simulink model "TurtlebotClosedLoop_template"  (R2023b)
settings: Solver=VariableStepAuto  StartTime=0.0  StopTime=150  MaxStep=0.1  RelTol=1e-3
undefined symbols (not defined in the file): q0
libraries: slpidlib x2, robotcorelib x1, robotmobilelib x1
settings Model: Creator=tpoggi  LastModifiedBy=jonpe

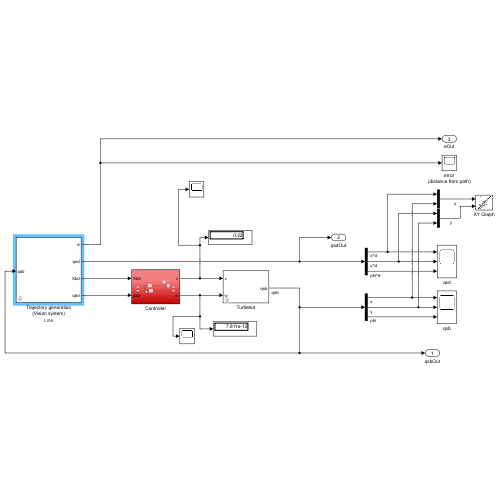
[thumbnail: Simulink's stored preview of the top-level diagram]
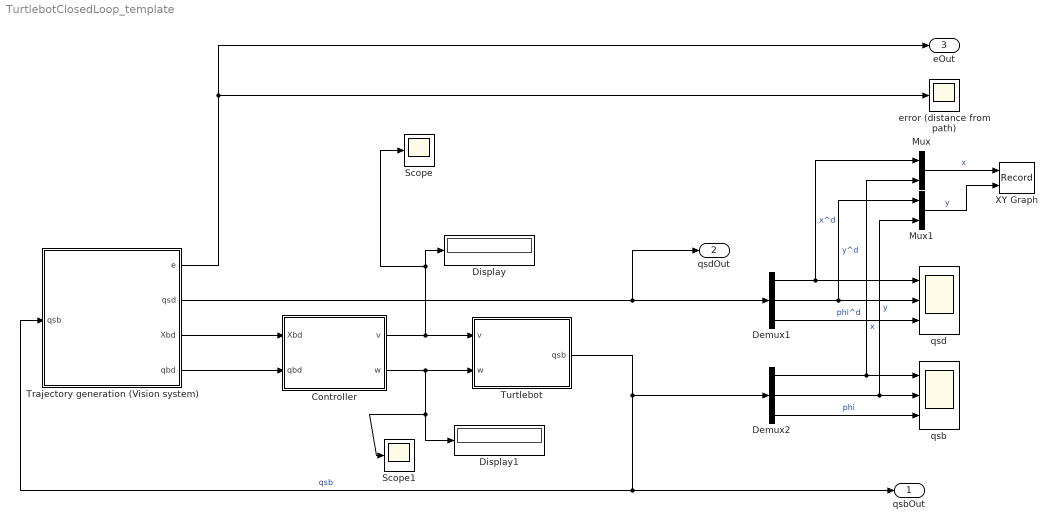
== system TurtlebotClosedLoop_template ==
  Controller : Subsystem
  Demux1 : Demux  Outputs=3
  Demux2 : Demux  Outputs=3
  Display : Display
  Display1 : Display
  Mux : Mux  Inputs=2
  Mux1 : Mux  Inputs=2
  Scope : Scope
  Scope1 : Scope
  Trajectory generation (Vision system) : Subsystem  mask(Description){PathType=Circle}
      mask prompts: PathType "Type of path"
      mask help:
      | Generate a trajectory by simulating a vision system that detects a path.
      | The path can be chosen to be a circle (radius=5m) or a straight line (y=x).
      |
      | Input:
      | - qsb: Configuration vector of the turtlebot qsb=[x,y,phi]
      |
      | Outputs:
      | - e: Error calculated as Euclidean distance with respect to the path (to be used only for visualisation).
      | - qsd: Desired trajectory in space frame (to be used only for visualisation).
      | - Xbd: SE(3) configuration of the desired position in the trurtlebot body frame.
      | - qbd: Minimal set of coordinates representing the point D on the path in the {b} frame.
      settings: AttributesFormatString=%<PathType>
      mask TypeOptions PathType: Trajectory Space Frame/PathType
  Turtlebot : Subsystem  mask{InitialState=q0}
      mask prompts: InitialState "robotics:robotslmobile:sharedblockmask:InitialStatePrompt"
      mask help:
      | Simple model of a turtlebot.
      |
      | Inputs:
      | - v: Linear velocity [m/s]
      | - w: Angular velocity [rad/s]
      |
      | Outputs:
      | - q: Configuration vector [x,y,phi]
      mask TypeOptions InitialState: Differential Drive Kinematic Model/InitialState
      mask DialogControl DescGroupVar Prompt: Description
      mask DialogControl ParameterGroupVar Prompt: Parameters:
      mask DialogControl InitialState Prompt: Initial state:
  XY Graph : Record  FileSettingsInternal="{\"entries\":[{\"content\":{\"excelSettings\":{\"content\":{},\"type\":\"Streamout.ExcelSettings\"}},\"type\":\"Streamout.FileSettingStorage\",\"uuid\":\"\"}],\"packageUris\":[\"http:\\/\\/schema.mathworks.com\\/mf0\\/streamout_blocks\\/R2020a\"],\"version\":\"1.0\"}"  Layout=[1 1]  SignalsInternal="{\"entries\":[{\"content\":{\"signals\":[{\"content\":{\"blockPath\":[],\"dimensions\":[2],\"domain\":\"\",\"hasChildren\":true,\"lineColor\":\"#139fff\",\"port\":1,\"sid\":[\"\"],\"signalID\":1,\"signalName\":\"x\"},\"type\":\"RecordBlkView.Signal\",\"uuid\":\"\"},{\"content\":{\"blockPath\":[],\"channel\":[1],\"dimensions\":[2],\"domain\":\"\",\"lineColor\":\"#4dbeee\",\"parentID\":1,\"plots\":[ 1 ],\"port\":1,\"sid\":[\"\"],\"signalID\":2,\"signalName\":\"x\"},\"type\":\"RecordBlkView.Signal\",\"uuid\":\"\"},{\"content\":{\"blockPath\":[],\"dimensions\":[2],\"domain\":\"\",\"hasChildren\":true,\"lineColor\":\"#b746ff\",\"port\":2,\"sid\":[\"\"],\"signalID\":3,\"signalName\":\"y\"},\"type\":\"RecordBlkView.Signal\",\"uuid\":\"\"},{\"content\":{\"blockPath\":[],\"channel\":[1],\"dimensions\":[2],\"domain\":\"\",\"lineColor\":\"#139fff\",\"parentID\":3,\"plots\":[ 1 ],\"port\":2,\"sid\":[\"\"],\"signalID\":4,\"signalName\":\"y\"},\"type\":\"RecordBlkView.Signal\",\"uuid\":\"\"},{\"content\":{\"blockPath\":[],\"channel\":[2],\"dimensions\":[2],\"domain\":\"\",\"lineColor\":\"#64d413\",\"parentID\":1,\"plots\":[ 1 ],\"port\":1,\"sid\":[\"\"],\"signalID\":5,\"signalName\":\"x\"},\"type\":\"RecordBlkView.Signal\",\"uuid\":\"\"},{\"content\":{\"blockPath\":[],\"channel\":[2],\"dimensions\":[2],\"domain\":\"\",\"lineColor\":\"#ff13a6\",\"parentID\":3,\"plots\":[ 1 ],\"port\":2,\"sid\":[\"\"],\"signalID\":6,\"signalName\":\"y\"},\"type\":\"RecordBlkView.Signal\",\"uuid\":\"\"}]},\"type\":\"RecordBlkView.InputSignals\",\"uuid\":\"\"}],\"packageUris\":[\"http:\\/\\/schema.mathworks.com\\/mf0\\/streamout_blocks\\/R2020a\"],\"version\":\"1.0\"}"  VisualizationBindings="{\"xyplotplugin\":{\"info\":[{\"series\":[{\"bindingParametersList\":[{\"parameter\":\"X-Axis\",\"signalID\":2,\"signalName\":\"x(1)\"},{\"parameter\":\"Y-Axis\",\"signalID\":4,\"signalName\":\"y(1)\"}],\"seriesID\":0},{\"bindingParametersList\":[{\"parameter\":\"X-Axis\",\"signalID\":5,\"signalName\":\"x(2)\"},{\"parameter\":\"Y-Axis\",\"signalID\":6,\"signalName\":\"y(2)\"}],\"seriesID\":1}],\"subplotID\":1}]}}"  CompatibilityTag=XY
  error (distance from path) : Scope
  qsb : Scope  NumInputPorts=3
  qsd : Scope  NumInputPorts=3
  qsbOut : Outport
  qsdOut : Outport  Port=2
  eOut : Outport  Port=3
  wires:
  Trajectory generation (Vision system)/1(e) -> eOut/1, error (distance from path)/1
  Demux2/2 -> qsb/2, Mux1/2  "y"
  Demux2/3 -> qsb/3  "phi"
  Mux1/1 -> XY Graph/2  "y"
  Trajectory generation (Vision system)/2(qsd) -> qsdOut/1, Demux1/1
  Mux/1 -> XY Graph/1  "x"
  Demux2/1 -> qsb/1, Mux/2  "x"
  Demux1/1 -> qsd/1, Mux/1  "x^d"
  Demux1/2 -> Mux1/1, qsd/2  "y^d"
  Turtlebot/1(qsb) -> Trajectory generation (Vision system)/1(qsb), qsbOut/1, Demux2/1  "qsb"
  Demux1/3 -> qsd/3  "phi^d"
  Trajectory generation (Vision system)/3(Xbd) -> Controller/1(Xbd)
  Trajectory generation (Vision system)/4(qbd) -> Controller/2(qbd)
  Controller/1(v) -> Scope/1, Display/1, Turtlebot/1(v)
  Controller/2(w) -> Scope1/1, Display1/1, Turtlebot/2(w)

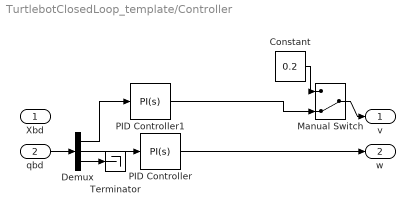
== system TurtlebotClosedLoop_template/Controller ==
  Xbd : Inport
  qbd : Inport  Port=2
  Constant : Constant  Value=0.2
  Demux : Demux  Outputs=3
  Manual Switch : ManualSwitch  CurrentSetting=0
  PID Controller : slpidlib/PID Controller  Controller=PI  Form=Parallel  TimeDomain=Continuous-time  UseExternalTs=off  SampleTime=-1  IntegratorMethod=Forward Euler  FilterMethod=Forward Euler  ControllerParametersSource=internal  P=2.5  I=1.25  UseKiTs=off  D=0  N=100  UseFilter=on  TunerSelectOption=Transfer Function Based (PID Tuner App)  InitialConditionSource=internal  InitialConditionForIntegrator=0  InitialConditionForFilter=0  DifferentiatorICPrevScaledInput=0  ExternalReset=none  TrackingMode=off  Kt=1  LimitOutput=on  SatLimitsSource=internal  UpperSaturationLimit=2.84  LowerSaturationLimit=-2.84  LinearizeAsGain=on  AntiWindupMode=clamping  Kb=1  LimitIntegrator=off  UpperIntegratorSaturationLimit=inf  LowerIntegratorSaturationLimit=-inf  POutMin=[]  POutMax=[]  IOutMin=[]  IOutMax=[]  DOutMin=[]  DOutMax=[]  NOutMin=[]  NOutMax=[]  SumOutMin=[]  SumOutMax=[]  SaturationOutMin=[]  SaturationOutMax=[]  PParamMin=[]  PParamMax=[]  IParamMin=[]  IParamMax=[]  DParamMin=[]  DParamMax=[]  NParamMin=[]  NParamMax=[]  KbParamMin=[]  KbParamMax=[]  KtParamMin=[]  KtParamMax=[]  KbOutMin=[]  KbOutMax=[]  KtOutMin=[]  KtOutMax=[]  IntegratorOutMin=[]  IntegratorOutMax=[]  FilterOutMin=[]  FilterOutMax=[]  SumI1OutMin=[]  SumI1OutMax=[]  SumI2OutMin=[]  SumI2OutMax=[]  SumI3OutMin=[]  SumI3OutMax=[]  SumI4OutMin=[]  SumI4OutMax=[]  SumDOutMin=[]  SumDOutMax=[]  DifferentiatorOutMin=[]  DifferentiatorOutMax=[]  FilterDiffOutCoefMin=[]  FilterDiffOutCoefMax=[]  ReciprocalOutMin=[]  ReciprocalOutMax=[]  SumDenOutMin=[]  SumDenOutMax=[]  SumNumOutMin=[]  SumNumOutMax=[]  DivideOutMin=[]  DivideOutMax=[]  UdiffTsProdOutMin=[]  UdiffTsProdOutMax=[]  NTsProdOutMin=[]  NTsProdOutMax=[]  UintegralTsProdOutMin=[]  UintegralTsProdOutMax=[]  UngainTsProdOutMin=[]  UngainTsProdOutMax=[]  ClampingZeroOutDataTypeStr=Inherit: Inherit via back propagation  ClampingZeroOutMin=[]  ClampingZeroOutMax=[]  FilterDenConstantOutDataTypeStr=Inherit: Inherit via back propagation  FilterDenConstantOutMin=[]  FilterDenConstantOutMax=[]  PCopyOutDataTypeStr=Inherit: Inherit via back propagation  PCopyOutMin=[]  PCopyOutMax=[]  NCopyOutDataTypeStr=Inherit: Inherit via back propagation  NCopyOutMin=[]  NCopyOutMax=[]  IntegratorContinuousStateAttributes=''  IntegratorStateMustResolveToSignalObject=off  IntegratorRTWStateStorageClass=Auto  FilterContinuousStateAttributes=''  FilterStateMustResolveToSignalObject=off  FilterRTWStateStorageClass=Auto  ParallelPVariant=InternalParameters  IdealPVariant=Disabled  IVariant=InternalParameters  DVariant=Disabled  IntegratorVariant=Continuous  SatVariant=Enabled  AWVariant=ContClampingParallel  PCopyVariant=Disabled  TRVariant=Disabled  FdbkBlocksVariant=Forward  IdealPFdbkVariant=Disabled  SatFdbkVariant=Disabled  DerivativeFilterVariant=Disabled  NVariant=Disabled  NCopyVariant=Disabled_SignalSpec  FilterICVariant=Disabled  IntegratorICVariant=InternalICs  ExternalResetVariant=Disabled  TRSumVariant=Passthrough  SumFdbkVariant=Disabled  SumVariant=Sum_PI  TsampFilterVariant=InternalTs  TsampNgainVariant=Passthrough  TsampIntegralVariant=Disabled_SignalSpec  ExternalSaturationOutDataTypeStr=Inherit: Same as second input
  PID Controller1 : slpidlib/PID Controller  Controller=PI  Form=Parallel  TimeDomain=Continuous-time  UseExternalTs=off  SampleTime=-1  IntegratorMethod=Forward Euler  FilterMethod=Forward Euler  ControllerParametersSource=internal  P=2.5  I=1.25  UseKiTs=off  D=0.25  N=100  UseFilter=on  TunerSelectOption=Transfer Function Based (PID Tuner App)  InitialConditionSource=internal  InitialConditionForIntegrator=0  InitialConditionForFilter=0  DifferentiatorICPrevScaledInput=0  ExternalReset=none  TrackingMode=off  Kt=1  LimitOutput=on  SatLimitsSource=internal  UpperSaturationLimit=0.22  LowerSaturationLimit=-0.22  LinearizeAsGain=on  AntiWindupMode=clamping  Kb=1  LimitIntegrator=off  UpperIntegratorSaturationLimit=inf  LowerIntegratorSaturationLimit=-inf  POutMin=[]  POutMax=[]  IOutMin=[]  IOutMax=[]  DOutMin=[]  DOutMax=[]  NOutMin=[]  NOutMax=[]  SumOutMin=[]  SumOutMax=[]  SaturationOutMin=[]  SaturationOutMax=[]  PParamMin=[]  PParamMax=[]  IParamMin=[]  IParamMax=[]  DParamMin=[]  DParamMax=[]  NParamMin=[]  NParamMax=[]  KbParamMin=[]  KbParamMax=[]  KtParamMin=[]  KtParamMax=[]  KbOutMin=[]  KbOutMax=[]  KtOutMin=[]  KtOutMax=[]  IntegratorOutMin=[]  IntegratorOutMax=[]  FilterOutMin=[]  FilterOutMax=[]  SumI1OutMin=[]  SumI1OutMax=[]  SumI2OutMin=[]  SumI2OutMax=[]  SumI3OutMin=[]  SumI3OutMax=[]  SumI4OutMin=[]  SumI4OutMax=[]  SumDOutMin=[]  SumDOutMax=[]  DifferentiatorOutMin=[]  DifferentiatorOutMax=[]  FilterDiffOutCoefMin=[]  FilterDiffOutCoefMax=[]  ReciprocalOutMin=[]  ReciprocalOutMax=[]  SumDenOutMin=[]  SumDenOutMax=[]  SumNumOutMin=[]  SumNumOutMax=[]  DivideOutMin=[]  DivideOutMax=[]  UdiffTsProdOutMin=[]  UdiffTsProdOutMax=[]  NTsProdOutMin=[]  NTsProdOutMax=[]  UintegralTsProdOutMin=[]  UintegralTsProdOutMax=[]  UngainTsProdOutMin=[]  UngainTsProdOutMax=[]  ClampingZeroOutDataTypeStr=Inherit: Inherit via back propagation  ClampingZeroOutMin=[]  ClampingZeroOutMax=[]  FilterDenConstantOutDataTypeStr=Inherit: Inherit via back propagation  FilterDenConstantOutMin=[]  FilterDenConstantOutMax=[]  PCopyOutDataTypeStr=Inherit: Inherit via back propagation  PCopyOutMin=[]  PCopyOutMax=[]  NCopyOutDataTypeStr=Inherit: Inherit via back propagation  NCopyOutMin=[]  NCopyOutMax=[]  IntegratorContinuousStateAttributes=''  IntegratorStateMustResolveToSignalObject=off  IntegratorRTWStateStorageClass=Auto  FilterContinuousStateAttributes=''  FilterStateMustResolveToSignalObject=off  FilterRTWStateStorageClass=Auto  ParallelPVariant=InternalParameters  IdealPVariant=Disabled  IVariant=InternalParameters  DVariant=Disabled  IntegratorVariant=Continuous  SatVariant=Enabled  AWVariant=ContClampingParallel  PCopyVariant=Disabled  TRVariant=Disabled  FdbkBlocksVariant=Forward  IdealPFdbkVariant=Disabled  SatFdbkVariant=Disabled  DerivativeFilterVariant=Disabled  NVariant=Disabled  NCopyVariant=Disabled_SignalSpec  FilterICVariant=Disabled  IntegratorICVariant=InternalICs  ExternalResetVariant=Disabled  TRSumVariant=Passthrough  SumFdbkVariant=Disabled  SumVariant=Sum_PI  TsampFilterVariant=InternalTs  TsampNgainVariant=Passthrough  TsampIntegralVariant=Disabled_SignalSpec  ExternalSaturationOutDataTypeStr=Inherit: Same as second input
  Terminator : Terminator
  v : Outport
  w : Outport  Port=2
  wires:
  qbd/1 -> Demux/1
  Demux/2 -> PID Controller/1
  Demux/3 -> Terminator/1
  PID Controller1/1 -> Manual Switch/2
  Demux/1 -> PID Controller1/1
  PID Controller/1 -> w/1
  Constant/1 -> Manual Switch/1
  Manual Switch/1 -> v/1

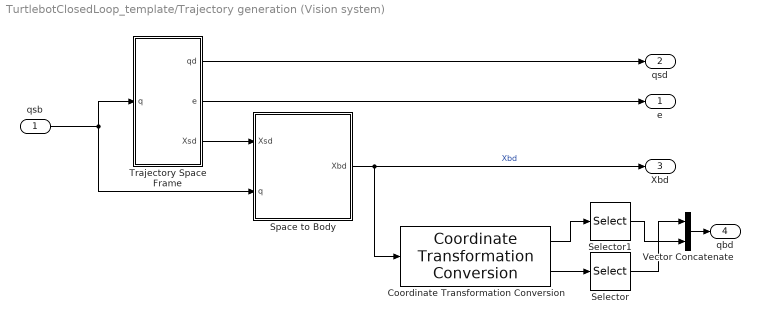
== system TurtlebotClosedLoop_template/Trajectory generation (Vision system) ==
  qsb : Inport
  Coordinate Transformation Conversion : robotcorelib/Coordinate Transformation Conversion  InputRepresentation=Homogeneous Transformation  InputEulerSequence=ZYX  ShowTrVecInputPort=on  OutputRepresentation=Euler Angles  OutputEulerSequence=ZYX  ShowTrVecOutputPort=on  SimulateUsing=Interpreted execution
  Selector : Selector  InputPortWidth=3  IndexOptions=Index vector (dialog)  Indices=[1 2]  OutputSizes=1
  Selector1 : Selector  InputPortWidth=3  IndexOptions=Index vector (dialog)  Indices=1  OutputSizes=1
  Space to Body : MATLAB Function  TreatAsAtomicUnit=on
  Trajectory Space Frame : Subsystem  mask{xr=0.3, yr=0, PathType=Circle, xc=0, yc=0, r=5, m=1, c=0}
      mask prompts: PathType "Type of path"; xc "Centre x coord"; yc "Centre y coord"; r "Radius"
      mask TypeOptions xr: Reference Point/xr/Value
      mask TypeOptions yr: Reference Point/yr/Value
      mask TypeOptions PathType: Distance from path/PathType | Find point on path/PathType
      mask TypeOptions xc: Distance from path/xc | Find point on path/xc
      mask TypeOptions yc: Distance from path/yc | Find point on path/yc
      mask TypeOptions r: Distance from path/r | Find point on path/r
      mask TypeOptions m: Distance from path/m | Find point on path/m
      mask TypeOptions c: Distance from path/c | Find point on path/c
      mask DialogControl ParameterGroupVar Prompt: Reference Point
      mask DialogControl Container4 Prompt: Line parameters
      mask DialogControl Container5 Prompt: Circle Paramters
  Vector Concatenate : Concatenate
  e : Outport
  qsd : Outport  Port=2
  Xbd : Outport  Port=3
  qbd : Outport  Port=4
  wires:
  qsb/1 -> Trajectory Space Frame/1(q), Space to Body/2(q)
  Space to Body/1(Xbd) -> Coordinate Transformation Conversion/1, Xbd/1  "Xbd"
  Trajectory Space Frame/1(qd) -> qsd/1
  Trajectory Space Frame/3(Xsd) -> Space to Body/1(Xsd)
  Trajectory Space Frame/2(e) -> e/1
  Coordinate Transformation Conversion/2 -> Selector/1
  Coordinate Transformation Conversion/1 -> Selector1/1
  Selector/1 -> Vector Concatenate/1
  Selector1/1 -> Vector Concatenate/2
  Vector Concatenate/1 -> qbd/1

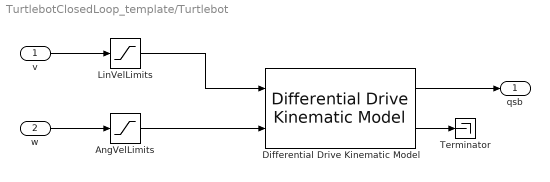
== system TurtlebotClosedLoop_template/Turtlebot ==
  v : Inport
  w : Inport  Port=2
  AngVelLimits : Saturate  UpperLimit=2.84  LowerLimit=-2.84
  Differential Drive Kinematic Model : robotmobilelib/Differential Drive Kinematic Model  VehicleInputs=Vehicle Speed & Heading Angular Velocity  WheelRadius=0.066  WheelSpeedRange=[-inf inf]  TrackWidth=0.16  InitialState=InitialState  SimulateUsing=Interpreted execution
  LinVelLimits : Saturate  UpperLimit=0.22  LowerLimit=-0.22
  Terminator : Terminator
  qsb : Outport
  wires:
  Differential Drive Kinematic Model/1 -> qsb/1
  v/1 -> LinVelLimits/1
  w/1 -> AngVelLimits/1
  Differential Drive Kinematic Model/2 -> Terminator/1
  LinVelLimits/1 -> Differential Drive Kinematic Model/1
  AngVelLimits/1 -> Differential Drive Kinematic Model/2

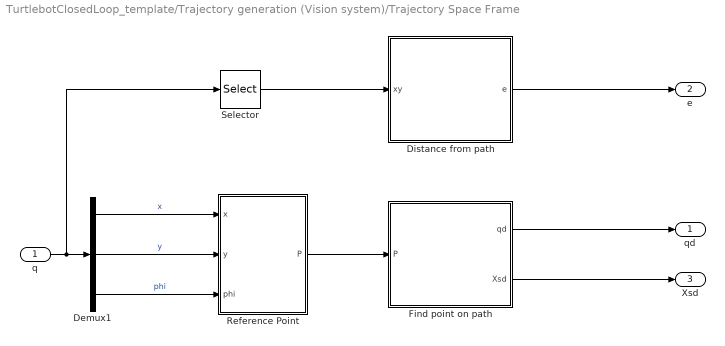
== system TurtlebotClosedLoop_template/Trajectory generation (Vision system)/Trajectory Space Frame ==
  q : Inport
  Demux1 : Demux  Outputs=3
  Distance from path : Subsystem  Variant=on  VariantControlMode=label  VariantControl=Circle  LabelModeActiveChoice=Circle  mask{PathType=Circle, xc=xc, yc=yc, r=r, m=m, c=c}
      mask prompts: PathType "Type of path"; xc "Centre x coord"; yc "Centre y coord"; r "Radius"
      mask TypeOptions PathType: LabelModeActiveChoice
      mask TypeOptions xc: Circle/xc/Value
      mask TypeOptions yc: Circle/yc/Value
      mask TypeOptions r: Circle/r/Value
      mask TypeOptions m: Line/m/Value
      mask TypeOptions c: Line/c/Value
      mask DialogControl Container4 Prompt: Circle parameters
      mask DialogControl Container3 Prompt: Line parameters
  Find point on path : Subsystem  Variant=on  VariantControlMode=label  VariantControl=Circle  LabelModeActiveChoice=Circle  mask(Paths){PathType=Circle, xc=xc, yc=yc, r=r, m=m, c=c}
      mask prompts: PathType "Type of path"; xc "Centre x coord:"; yc "Centre y coord"; r "Radius"
      mask help:
      | Two option are available:
      | 1) Straight line:
      | y=mx+c
      |
      | 2) Circle:
      | (x-xc)^2 + (y-yc)^2 = r
      mask TypeOptions PathType: LabelModeActiveChoice
      mask TypeOptions xc: Circle/xc/Value
      mask TypeOptions yc: Circle/yc/Value
      mask TypeOptions r: Circle/rx/Gain | Circle/ry/Gain
      mask TypeOptions m: Line/m/Value
      mask TypeOptions c: Line/c/Value
      mask DialogControl Container4 Prompt: Circle parameters
      mask DialogControl Container3 Prompt: Line parameters
  Reference Point : Subsystem
  Selector : Selector  InputPortWidth=3  IndexOptions=Index vector (dialog)  Indices=[1 2]  OutputSizes=1
  qd : Outport
  e : Outport  Port=2
  Xsd : Outport  Port=3
  wires:
  Demux1/2 -> Reference Point/2(y)  "y"
  q/1 -> Selector/1, Demux1/1
  Demux1/3 -> Reference Point/3(phi)  "phi"
  Demux1/1 -> Reference Point/1(x)  "x"
  Reference Point/1(P) -> Find point on path/1(P)
  Find point on path/1(qd) -> qd/1
  Find point on path/2(Xsd) -> Xsd/1
  Selector/1 -> Distance from path/1(xy)
  Distance from path/1(e) -> e/1

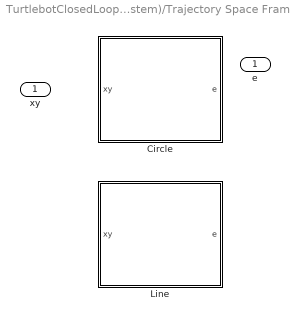
== system TurtlebotClosedLoop_template/Trajectory generation (Vision system)/Trajectory Space Frame/Distance from path ==
  xy : Inport
  Circle : Subsystem  VariantControl=Circle
  Line : Subsystem  VariantControl=Line
  e : Outport

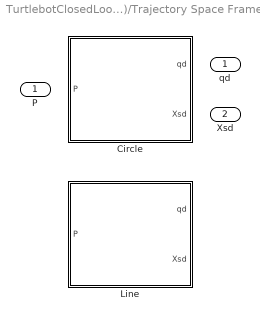
== system TurtlebotClosedLoop_template/Trajectory generation (Vision system)/Trajectory Space Frame/Find point on path ==
  P : Inport
  Circle : Subsystem  VariantControl=Circle
  Line : Subsystem  VariantControl=Line
  qd : Outport
  Xsd : Outport  Port=2

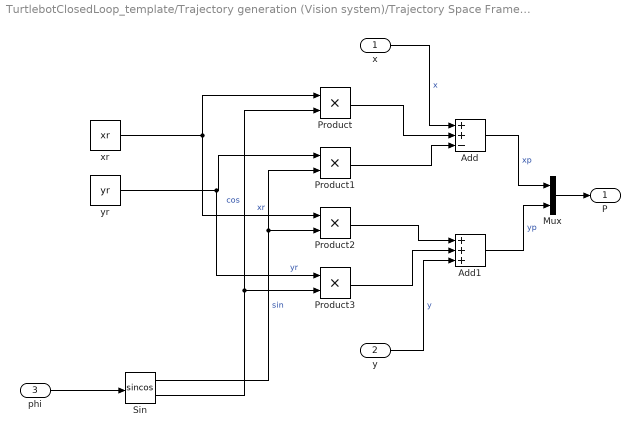
== system TurtlebotClosedLoop_template/Trajectory generation (Vision system)/Trajectory Space Frame/Reference Point ==
  x : Inport
  y : Inport  Port=2
  phi : Inport  Port=3
  Add : Sum  Inputs=++-
  Add1 : Sum  Inputs=+++
  Mux : Mux  Inputs=2
  Product{,1..3} (4 alike) : Product
  Sin : Trigonometry  Operator=sincos
  xr : Constant  Value=xr
  yr : Constant  Value=yr
  P : Outport
  wires:
  phi/1 -> Sin/1
  xr/1 -> Product2/1, Product/1  "xr"
  yr/1 -> Product3/1, Product1/1  "yr"
  Sin/2 -> Product3/2, Product/2  "cos"
  Sin/1 -> Product2/2, Product1/2  "sin"
  Product/1 -> Add/2
  Product1/1 -> Add/3
  Product2/1 -> Add1/1
  Product3/1 -> Add1/2
  Add/1 -> Mux/1  "xp"
  Add1/1 -> Mux/2  "yp"
  x/1 -> Add/1  "x"
  y/1 -> Add1/3  "y"
  Mux/1 -> P/1

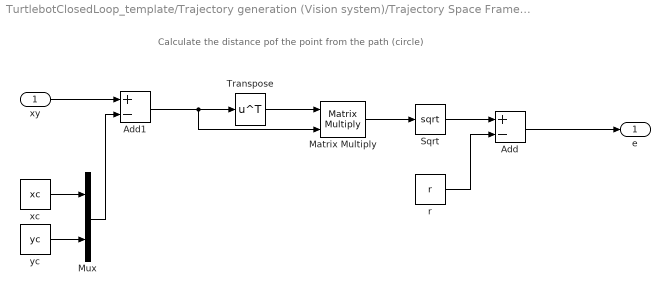
== system TurtlebotClosedLoop_template/Trajectory generation (Vision system)/Trajectory Space Frame/Distance from path/Circle ==
  note: Calculate the distance pof the point from the path (circle)
  xy : Inport
  Add : Sum  Inputs=+-
  Add1 : Sum  Inputs=+-
  Matrix Multiply : Product  Multiplication=Matrix(*)
  Mux : Mux  Inputs=2
  Sqrt : Sqrt
  Transpose : Math  Operator=transpose
  r : Constant  Value=r
  xc : Constant  Value=xc
  yc : Constant  Value=yc
  e : Outport
  wires:
  xy/1 -> Add1/1
  Transpose/1 -> Matrix Multiply/1
  Matrix Multiply/1 -> Sqrt/1
  Sqrt/1 -> Add/1
  r/1 -> Add/2
  Add/1 -> e/1
  Add1/1 -> Matrix Multiply/2, Transpose/1
  xc/1 -> Mux/1
  yc/1 -> Mux/2
  Mux/1 -> Add1/2

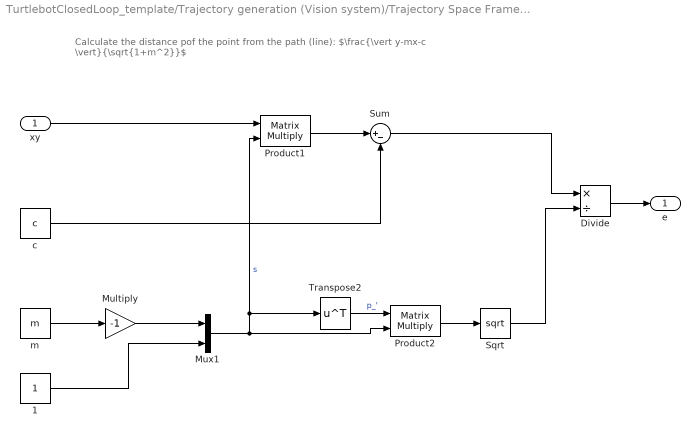
== system TurtlebotClosedLoop_template/Trajectory generation (Vision system)/Trajectory Space Frame/Distance from path/Line ==
  note: Calculate the distance pof the point from the path (line):
      | $\frac{\vert y-mx-c \vert}{\sqrt{1+m^2}}$
  xy : Inport
  1 : Constant
  Divide : Product  Inputs=*/
  Multiply : Gain  Gain=-1
  Mux1 : Mux  Inputs=2
  Product1 : Product  Multiplication=Matrix(*)
  Product2 : Product  Multiplication=Matrix(*)
  Sqrt : Sqrt
  Sum : Sum  Inputs=|+-
  Transpose2 : Math  Operator=transpose
  c : Constant  Value=c
  m : Constant  Value=m
  e : Outport
  wires:
  Mux1/1 -> Product2/2, Product1/2, Transpose2/1  "s"
  m/1 -> Multiply/1
  c/1 -> Sum/2
  xy/1 -> Product1/1
  Divide/1 -> e/1
  Transpose2/1 -> Product2/1  "p_'"
  Product2/1 -> Sqrt/1
  Product1/1 -> Sum/1
  Sum/1 -> Divide/1
  Sqrt/1 -> Divide/2
  Multiply/1 -> Mux1/1
  1/1 -> Mux1/2

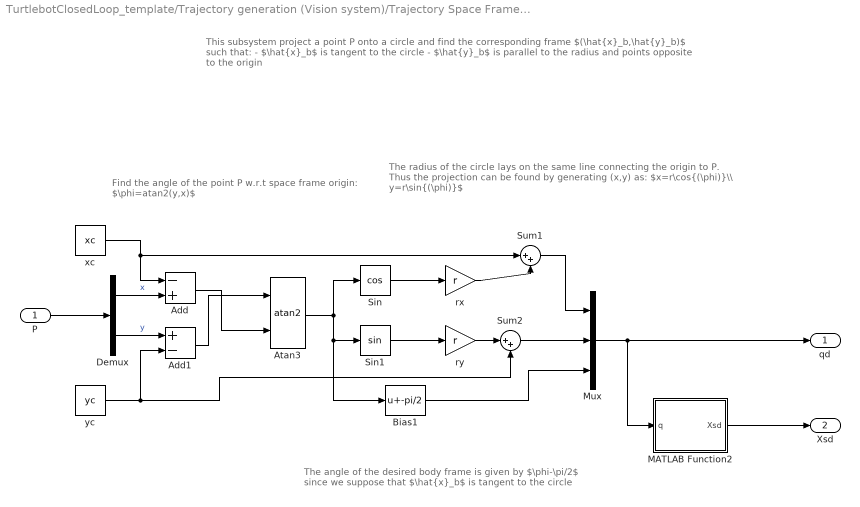
== system TurtlebotClosedLoop_template/Trajectory generation (Vision system)/Trajectory Space Frame/Find point on path/Circle ==
  note: This subsystem project a point P onto a circle and find the corresponding frame $(\hat{x}_b,\hat{y}_b)$
      | such that:
      | - $\hat{x}_b$ is tangent to the circle
      | - $\hat{y}_b$ is parallel to the radius and points opposite to the origin
  note: The angle of the desired body frame is given by $\phi-\pi/2$
      | since we suppose that $\hat{x}_b$ is tangent to the circle
  note: Find the angle of the point P w.r.t space frame origin:
      | $\phi=atan2(y,x)$
  note: The radius of the circle lays on the same line connecting the origin to P.
      | Thus the projection can be found by generating (x,y) as:
      | $x=r\cos{(\phi)}\\ y=r\sin{(\phi)}$
  P : Inport
  Add : Sum  Inputs=-+
  Add1 : Sum  Inputs=+-
  Atan3 : Trigonometry  Operator=atan2
  Bias1 : Bias  Bias=-pi/2  SaturateOnIntegerOverflow=off
  Demux : Demux  Outputs=2
  MATLAB Function2 : MATLAB Function  TreatAsAtomicUnit=on
  Mux : Mux  Inputs=3
  Sin : Trigonometry  Operator=cos
  Sin1 : Trigonometry
  Sum1 : Sum  Inputs=|++
  Sum2 : Sum  Inputs=|++
  rx : Gain  Gain=r
  ry : Gain  Gain=r
  xc : Constant  Value=xc
  yc : Constant  Value=yc
  qd : Outport
  Xsd : Outport  Port=2
  wires:
  Sin/1 -> rx/1
  Atan3/1 -> Sin/1, Bias1/1, Sin1/1
  Bias1/1 -> Mux/3
  MATLAB Function2/1(Xsd) -> Xsd/1
  P/1 -> Demux/1
  Demux/1 -> Add/2  "x"
  Sin1/1 -> ry/1
  Add1/1 -> Atan3/1
  Demux/2 -> Add1/1  "y"
  Add/1 -> Atan3/2
  Mux/1 -> qd/1, MATLAB Function2/1(q)
  xc/1 -> Sum1/1, Add/1
  yc/1 -> Sum2/2, Add1/2
  rx/1 -> Sum1/2
  Sum1/1 -> Mux/1
  Sum2/1 -> Mux/2
  ry/1 -> Sum2/1

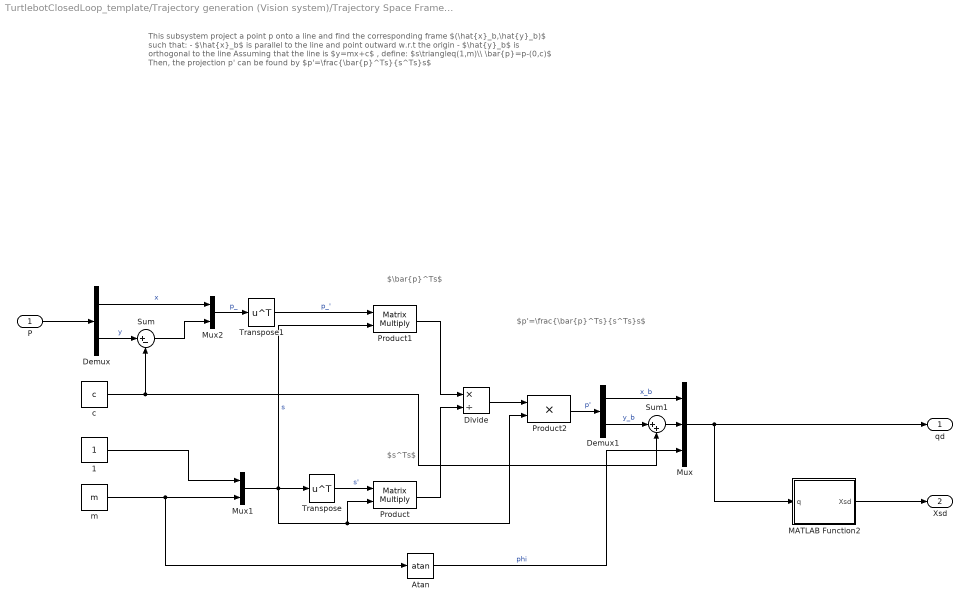
== system TurtlebotClosedLoop_template/Trajectory generation (Vision system)/Trajectory Space Frame/Find point on path/Line ==
  note: $p'=\frac{\bar{p}^Ts}{s^Ts}s$
  note: $\bar{p}^Ts$
  note: This subsystem project a point p onto a line and find the corresponding frame $(\hat{x}_b,\hat{y}_b)$
      | such that:
      | - $\hat{x}_b$ is parallel to the line and point outward w.r.t the origin
      | - $\hat{y}_b$ is orthogonal to the line
      |
      | Assuming that the line is $y=mx+c$ , define:
      | $s\triangleq(1,m)\\ \bar{p}=p-(0,c)$
      | Then, the projection p' can be found by
      | $p'=\frac{\bar{p}^Ts}{s^Ts}s$
  note: $s^Ts$
  P : Inport
  1 : Constant
  Atan : Trigonometry  Operator=atan
  Demux : Demux  Outputs=2
  Demux1 : Demux  Outputs=2
  Divide : Product  Inputs=*/
  MATLAB Function2 : MATLAB Function  TreatAsAtomicUnit=on
  Mux : Mux  Inputs=3
  Mux1 : Mux  Inputs=2
  Mux2 : Mux  Inputs=2
  Product : Product  Multiplication=Matrix(*)
  Product1 : Product  Multiplication=Matrix(*)
  Product2 : Product
  Sum : Sum  Inputs=|+-
  Sum1 : Sum  Inputs=|++
  Transpose : Math  Operator=transpose
  Transpose1 : Math  Operator=transpose
  c : Constant  Value=c
  m : Constant  Value=m
  qd : Outport
  Xsd : Outport  Port=2
  wires:
  Mux/1 -> MATLAB Function2/1(q), qd/1
  Demux/2 -> Sum/1  "y"
  Demux/1 -> Mux2/1  "x"
  P/1 -> Demux/1
  MATLAB Function2/1(Xsd) -> Xsd/1
  Atan/1 -> Mux/3  "phi"
  c/1 -> Sum1/2, Sum/2
  1/1 -> Mux1/1
  m/1 -> Atan/1, Mux1/2
  Sum/1 -> Mux2/2
  Mux1/1 -> Product2/2, Product/2, Product1/2, Transpose/1  "s"
  Mux2/1 -> Transpose1/1  "p_"
  Transpose/1 -> Product/1  "s'"
  Transpose1/1 -> Product1/1  "p_'"
  Product1/1 -> Divide/1
  Product/1 -> Divide/2
  Divide/1 -> Product2/1
  Product2/1 -> Demux1/1  "p'"
  Demux1/1 -> Mux/1  "x_b"
  Demux1/2 -> Sum1/1  "y_b"
  Sum1/1 -> Mux/2

== matlab function TurtlebotClosedLoop_template/Trajectory generation (Vision system)/Trajectory Space Frame/Find point on path/Circle/MATLAB Function2 ==
  data: Xsd output; q input
function Xsd = fcn(q)

Xsd=[cos(q(3)), -sin(q(3)), 0, q(1);
    sin(q(3)), cos(q(3)), 0, q(2);
    0,  0,  1,  0;
    0,  0,  0,  1];

== matlab function TurtlebotClosedLoop_template/Trajectory generation (Vision system)/Space to Body ==
  data: Xsd input; q input; Xbd output
function Xbd = ChangeFrame(Xsd, q)

Xsb=[cos(q(3)), -sin(q(3)), 0, q(1);
    sin(q(3)), cos(q(3)), 0, q(2);
    0,  0,  1,  0;
    0,  0,  0,  1];

Xbd= Xsb\Xsd;

== matlab function TurtlebotClosedLoop_template/Trajectory generation (Vision system)/Trajectory Space Frame/Find point on path/Line/MATLAB Function2 ==
  data: Xsd output; q input
function Xsd = fcn(q)

Xsd=[cos(q(3)), -sin(q(3)), 0, q(1);
    sin(q(3)), cos(q(3)), 0, q(2);
    0,  0,  1,  0;
    0,  0,  0,  1];
